simulink model "gm_gaussianFilter"  (R2024a)
settings: Solver=FixedStepDiscrete  StartTime=0.0  StopTime=1  RelTol=1e-3
undefined symbols (not defined in the file or in its folder): G
libraries: hdlsllib x33, simulink x27, visionsources x1, visionsinks x1
(part 2 of 2)

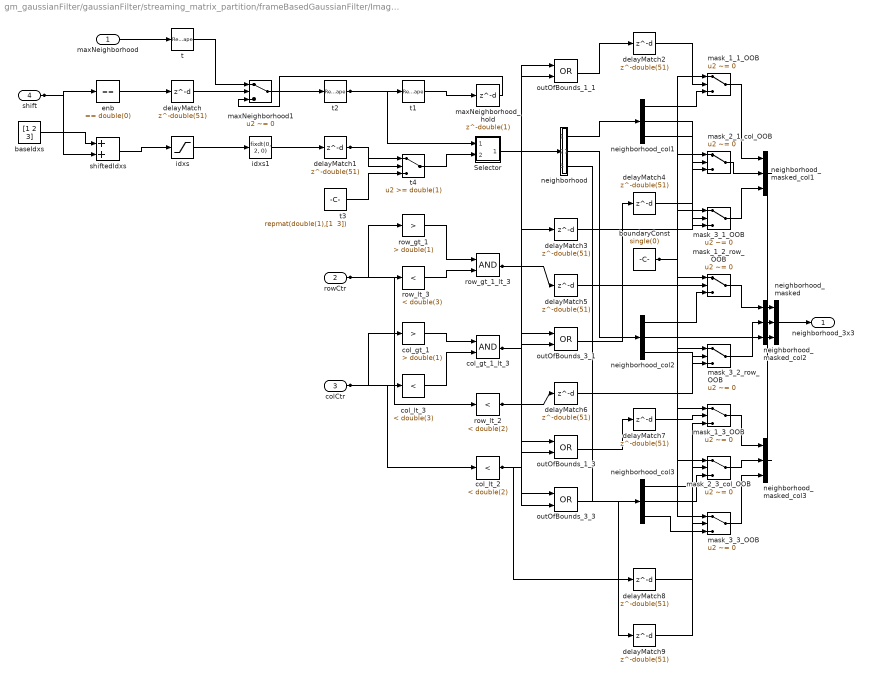
== system gm_gaussianFilter/gaussianFilter/streaming_matrix_partition/frameBasedGaussianFilter/ImageIn_NeighborhoodCreator/BoundaryCheck_3x3 ==
  maxNeighborhood : Inport  OutDataTypeStr=single  SampleTime=2.77039007092199e-06
  rowCtr : Inport  Port=2  OutDataTypeStr=fixdt(0,9,0,'DataTypeOverride', 'Off')  SampleTime=2.77039007092199e-06
  colCtr : Inport  Port=3  OutDataTypeStr=fixdt(0,10,0,'DataTypeOverride', 'Off')  SampleTime=2.77039007092199e-06
  shift : Inport  Port=4  OutDataTypeStr=fixdt(0,1,0,'DataTypeOverride', 'Off')  SampleTime=2.77039007092199e-06
  Selector : Subsystem
  baseIdxs : Constant  Value=[1 2 3]  OutDataTypeStr=fixdt(0, 2, 0)  SampleTime=2.77039007092199e-06
  boundaryConst : Constant  Value=single(0)  OutDataTypeStr=single  SampleTime=2.77039007092199e-06
  col_gt_1 : simulink/Logic and Bit Operations/Compare To Constant  relop=>  const=double(1)  OutDataTypeStr=boolean
  col_gt_1_lt_3 : Logic  AllPortsSameDT=off  OutDataTypeStr=boolean  SampleTime=2.77039007092199e-06
  col_lt_2 : simulink/Logic and Bit Operations/Compare To Constant  relop=<  const=double(2)  OutDataTypeStr=boolean
  col_lt_3 : simulink/Logic and Bit Operations/Compare To Constant  relop=<  const=double(3)  OutDataTypeStr=boolean
  delayMatch{,1..9} (10 alike) : Delay  DelayLength=double(51)  InitialCondition=0  SampleTime=2.77039007092199e-06
  enb : simulink/Logic and Bit Operations/Compare To Constant  relop===  const=double(0)  OutDataTypeStr=boolean
  idxs : Saturate  UpperLimit=double(3)  LowerLimit=double(1)  SampleTime=2.77039007092199e-06  OutDataTypeStr=fixdt(0, 3, 0)
  idxs1 : DataTypeConversion  OutDataTypeStr=fixdt(0, 2, 0)  SampleTime=2.77039007092199e-06  SaturateOnIntegerOverflow=off  RndMeth=Floor
  mask_1_1_OOB : Switch  Criteria=u2 ~= 0  Threshold=double(0)  OutDataTypeStr=single  SampleTime=2.77039007092199e-06  SaturateOnIntegerOverflow=off  InputSameDT=off
  mask_1_2_row_OOB : Switch  Criteria=u2 ~= 0  Threshold=double(0)  OutDataTypeStr=single  SampleTime=2.77039007092199e-06  SaturateOnIntegerOverflow=off  InputSameDT=off
  mask_1_3_OOB : Switch  Criteria=u2 ~= 0  Threshold=double(0)  OutDataTypeStr=single  SampleTime=2.77039007092199e-06  SaturateOnIntegerOverflow=off  InputSameDT=off
  mask_2_1_col_OOB : Switch  Criteria=u2 ~= 0  Threshold=double(0)  OutDataTypeStr=single  SampleTime=2.77039007092199e-06  SaturateOnIntegerOverflow=off  InputSameDT=off
  mask_2_3_col_OOB : Switch  Criteria=u2 ~= 0  Threshold=double(0)  OutDataTypeStr=single  SampleTime=2.77039007092199e-06  SaturateOnIntegerOverflow=off  InputSameDT=off
  mask_3_1_OOB : Switch  Criteria=u2 ~= 0  Threshold=double(0)  OutDataTypeStr=single  SampleTime=2.77039007092199e-06  SaturateOnIntegerOverflow=off  InputSameDT=off
  mask_3_2_row_OOB : Switch  Criteria=u2 ~= 0  Threshold=double(0)  OutDataTypeStr=single  SampleTime=2.77039007092199e-06  SaturateOnIntegerOverflow=off  InputSameDT=off
  mask_3_3_OOB : Switch  Criteria=u2 ~= 0  Threshold=double(0)  OutDataTypeStr=single  SampleTime=2.77039007092199e-06  SaturateOnIntegerOverflow=off  InputSameDT=off
  maxNeighborhood1 : Switch  Criteria=u2 ~= 0  Threshold=double(0)  OutDataTypeStr=single  SampleTime=2.77039007092199e-06  SaturateOnIntegerOverflow=off  InputSameDT=off
  maxNeighborhood_hold : Delay  DelayLength=double(1)  InitialCondition=0  SampleTime=2.77039007092199e-06
  neighborhood : Subsystem
  neighborhood_col1 : Demux  Outputs=3
  neighborhood_col2 : Demux  Outputs=3
  neighborhood_col3 : Demux  Outputs=3
  neighborhood_masked : Concatenate  NumInputs=3  Mode=Multidimensional array  ConcatenateDimension=2
  neighborhood_masked_col1 : Concatenate  NumInputs=3  Mode=Multidimensional array
  neighborhood_masked_col2 : Concatenate  NumInputs=3  Mode=Multidimensional array
  neighborhood_masked_col3 : Concatenate  NumInputs=3  Mode=Multidimensional array
  outOfBounds_1_1 : Logic  Operator=OR  AllPortsSameDT=off  OutDataTypeStr=boolean  SampleTime=2.77039007092199e-06
  outOfBounds_1_3 : Logic  Operator=OR  AllPortsSameDT=off  OutDataTypeStr=boolean  SampleTime=2.77039007092199e-06
  outOfBounds_3_1 : Logic  Operator=OR  AllPortsSameDT=off  OutDataTypeStr=boolean  SampleTime=2.77039007092199e-06
  outOfBounds_3_3 : Logic  Operator=OR  AllPortsSameDT=off  OutDataTypeStr=boolean  SampleTime=2.77039007092199e-06
  row_gt_1 : simulink/Logic and Bit Operations/Compare To Constant  relop=>  const=double(1)  OutDataTypeStr=boolean
  row_gt_1_lt_3 : Logic  AllPortsSameDT=off  OutDataTypeStr=boolean  SampleTime=2.77039007092199e-06
  row_lt_2 : simulink/Logic and Bit Operations/Compare To Constant  relop=<  const=double(2)  OutDataTypeStr=boolean
  row_lt_3 : simulink/Logic and Bit Operations/Compare To Constant  relop=<  const=double(3)  OutDataTypeStr=boolean
  shiftedIdxs : Sum  OutDataTypeStr=fixdt(0, 3, 0)  SampleTime=2.77039007092199e-06
  t : Reshape  OutputDimensionality=Column vector (2-D)
  t1 : Reshape  OutputDimensionality=Column vector (2-D)
  t2 : Reshape  OutputDimensionality=Customize  OutputDimensions=[3,3]
  t3 : Constant  Value="repmat(double(1),[1  3])"  OutDataTypeStr=fixdt(0, 2, 0)  SampleTime=2.77039007092199e-06
  t4 : Switch  Threshold=double(1)  OutDataTypeStr=fixdt(0, 2, 0)  SampleTime=2.77039007092199e-06  SaturateOnIntegerOverflow=off  InputSameDT=off
  neighborhood_3x3 : Outport  OutDataTypeStr=single  SampleTime=2.77039007092199e-06
  wires:
  maxNeighborhood/1 -> t/1
  rowCtr/1 -> row_lt_2/1, row_lt_3/1, row_gt_1/1
  colCtr/1 -> col_lt_2/1, col_lt_3/1, col_gt_1/1
  shift/1 -> shiftedIdxs/2, enb/1
  delayMatch/1 -> maxNeighborhood1/2
  baseIdxs/1 -> shiftedIdxs/1
  shiftedIdxs/1 -> idxs/1
  idxs/1 -> idxs1/1
  delayMatch1/1 -> t4/2, t4/1
  Selector/1(Out1) -> neighborhood/1(in0)
  boundaryConst/1 -> mask_3_3_OOB/1, mask_3_2_row_OOB/1, mask_3_1_OOB/1, mask_2_3_col_OOB/1, mask_2_1_col_OOB/1, mask_1_3_OOB/1, mask_1_2_row_OOB/1, mask_1_1_OOB/1
  neighborhood_col1/1 -> mask_1_1_OOB/3
  neighborhood_col2/1 -> mask_1_2_row_OOB/3
  neighborhood_col3/1 -> mask_1_3_OOB/3
  neighborhood_col1/2 -> mask_2_1_col_OOB/3
  neighborhood_col2/2 -> neighborhood_masked_col2/2
  neighborhood_col3/2 -> mask_2_3_col_OOB/3
  neighborhood_col1/3 -> mask_3_1_OOB/3
  neighborhood_col2/3 -> mask_3_2_row_OOB/3
  neighborhood_col3/3 -> mask_3_3_OOB/3
  neighborhood/1(out0) -> neighborhood_col1/1
  neighborhood/2(out1) -> neighborhood_col2/1
  neighborhood/3(out2) -> neighborhood_col3/1
  row_gt_1/1 -> row_gt_1_lt_3/1
  row_lt_3/1 -> row_gt_1_lt_3/2
  delayMatch5/1 -> mask_1_2_row_OOB/2
  col_gt_1/1 -> col_gt_1_lt_3/1
  col_lt_3/1 -> col_gt_1_lt_3/2
  delayMatch3/1 -> mask_2_1_col_OOB/2
  delayMatch2/1 -> mask_1_1_OOB/2
  mask_1_1_OOB/1 -> neighborhood_masked_col1/1
  mask_1_2_row_OOB/1 -> neighborhood_masked_col2/1
  delayMatch8/1 -> mask_2_3_col_OOB/2
  delayMatch7/1 -> mask_1_3_OOB/2
  mask_1_3_OOB/1 -> neighborhood_masked_col3/1
  mask_2_1_col_OOB/1 -> neighborhood_masked_col1/2
  mask_2_3_col_OOB/1 -> neighborhood_masked_col3/2
  delayMatch6/1 -> mask_3_2_row_OOB/2
  delayMatch4/1 -> mask_3_1_OOB/2
  mask_3_1_OOB/1 -> neighborhood_masked_col1/3
  mask_3_2_row_OOB/1 -> neighborhood_masked_col2/3
  delayMatch9/1 -> mask_3_3_OOB/2
  mask_3_3_OOB/1 -> neighborhood_masked_col3/3
  neighborhood_masked/1 -> neighborhood_3x3/1
  neighborhood_masked_col1/1 -> neighborhood_masked/1
  neighborhood_masked_col2/1 -> neighborhood_masked/2
  neighborhood_masked_col3/1 -> neighborhood_masked/3
  t/1 -> maxNeighborhood1/1
  enb/1 -> delayMatch/1
  idxs1/1 -> delayMatch1/1
  outOfBounds_1_1/1 -> delayMatch2/1
  col_gt_1_lt_3/1 -> delayMatch3/1, outOfBounds_3_1/2, outOfBounds_1_1/2
  outOfBounds_3_1/1 -> delayMatch4/1
  row_gt_1_lt_3/1 -> delayMatch5/1, outOfBounds_1_3/1, outOfBounds_1_1/1
  row_lt_2/1 -> delayMatch6/1, outOfBounds_3_3/1, outOfBounds_3_1/1
  outOfBounds_1_3/1 -> delayMatch7/1
  col_lt_2/1 -> delayMatch8/1, outOfBounds_3_3/2, outOfBounds_1_3/2
  outOfBounds_3_3/1 -> delayMatch9/1
  t2/1 -> t1/1, Selector/1(In1)
  t1/1 -> maxNeighborhood_hold/1
  maxNeighborhood_hold/1 -> maxNeighborhood1/3
  maxNeighborhood1/1 -> t2/1
  t3/1 -> t4/3
  t4/1 -> Selector/2(In2)

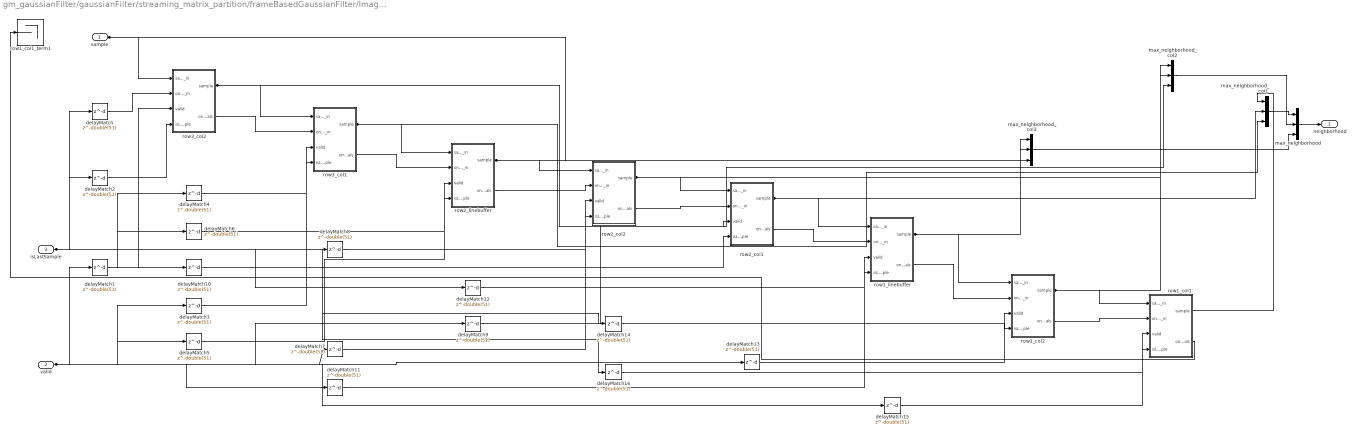
== system gm_gaussianFilter/gaussianFilter/streaming_matrix_partition/frameBasedGaussianFilter/ImageIn_NeighborhoodCreator/NeighborhoodCreator_3x3 ==
  sample : Inport  OutDataTypeStr=single  SampleTime=2.77039007092199e-06
  valid : Inport  Port=2  OutDataTypeStr=boolean  SampleTime=2.77039007092199e-06
  isLastSample : Inport  Port=3  OutDataTypeStr=boolean  SampleTime=2.77039007092199e-06
  delayMatch{,1..16} (17 alike) : Delay  DelayLength=double(51)  InitialCondition=0  SampleTime=2.77039007092199e-06
  max_neighborhood : Concatenate  NumInputs=3  Mode=Multidimensional array  ConcatenateDimension=2
  max_neighborhood_col1 : Concatenate  NumInputs=3  Mode=Multidimensional array
  max_neighborhood_col2 : Concatenate  NumInputs=3  Mode=Multidimensional array
  max_neighborhood_col3 : Concatenate  NumInputs=3  Mode=Multidimensional array
  row1_col1 : Subsystem
  row1_col1_term1 : Terminator
  row1_col2 : Subsystem
  row1_linebuffer : Subsystem
  row2_col1 : Subsystem
  row2_col2 : Subsystem
  row2_linebuffer : Subsystem
  row3_col1 : Subsystem
  row3_col2 : Subsystem
  neighborhood : Outport  OutDataTypeStr=single  SampleTime=2.77039007092199e-06
  wires:
  sample/1 -> max_neighborhood_col3/3, row3_col2/1(sample_in)
  delayMatch1/1 -> row3_col2/3(valid)
  delayMatch/1 -> row3_col2/2(onEndVals_in)
  row3_col2/1(sample) -> max_neighborhood_col2/3, row3_col1/1(sample_in)
  row3_col2/2(onEndVals) -> row3_col1/2(onEndVals_in)
  row3_col1/1(sample) -> max_neighborhood_col1/3, row2_linebuffer/1(sample_in)
  row3_col1/2(onEndVals) -> row2_linebuffer/2(onEndVals_in)
  row2_linebuffer/1(sample) -> max_neighborhood_col3/2, row2_col2/1(sample_in)
  row2_linebuffer/2(onEndVals) -> row2_col2/2(onEndVals_in)
  row2_col2/1(sample) -> max_neighborhood_col2/2, row2_col1/1(sample_in)
  row2_col2/2(onEndVals) -> row2_col1/2(onEndVals_in)
  row2_col1/1(sample) -> max_neighborhood_col1/2, row1_linebuffer/1(sample_in)
  row2_col1/2(onEndVals) -> row1_linebuffer/2(onEndVals_in)
  row1_linebuffer/1(sample) -> max_neighborhood_col3/1, row1_col2/1(sample_in)
  row1_linebuffer/2(onEndVals) -> row1_col2/2(onEndVals_in)
  row1_col2/1(sample) -> max_neighborhood_col2/1, row1_col1/1(sample_in)
  row1_col2/2(onEndVals) -> row1_col1/2(onEndVals_in)
  row1_col1/1(sample) -> max_neighborhood_col1/1
  row1_col1/2(onEndVals) -> row1_col1_term1/1
  max_neighborhood/1 -> neighborhood/1
  max_neighborhood_col1/1 -> max_neighborhood/1
  max_neighborhood_col2/1 -> max_neighborhood/2
  max_neighborhood_col3/1 -> max_neighborhood/3
  delayMatch2/1 -> row3_col2/4(isLastSample)
  delayMatch3/1 -> row3_col1/3(valid)
  delayMatch4/1 -> row3_col1/4(isLastSample)
  delayMatch5/1 -> row2_linebuffer/3(valid)
  delayMatch6/1 -> row2_linebuffer/4(isLastSample)
  delayMatch7/1 -> row2_col2/3(valid)
  delayMatch8/1 -> row2_col2/4(isLastSample)
  delayMatch9/1 -> row2_col1/3(valid)
  delayMatch10/1 -> row2_col1/4(isLastSample)
  delayMatch11/1 -> row1_linebuffer/3(valid)
  delayMatch12/1 -> row1_linebuffer/4(isLastSample)
  delayMatch13/1 -> row1_col2/3(valid)
  delayMatch14/1 -> row1_col2/4(isLastSample)
  delayMatch15/1 -> row1_col1/3(valid)
  delayMatch16/1 -> row1_col1/4(isLastSample)
  valid/1 -> delayMatch15/1, delayMatch13/1, delayMatch11/1, delayMatch9/1, delayMatch7/1, delayMatch5/1, delayMatch3/1, delayMatch1/1
  isLastSample/1 -> delayMatch16/1, delayMatch14/1, delayMatch12/1, delayMatch10/1, delayMatch8/1, delayMatch6/1, delayMatch4/1, delayMatch2/1, delayMatch/1

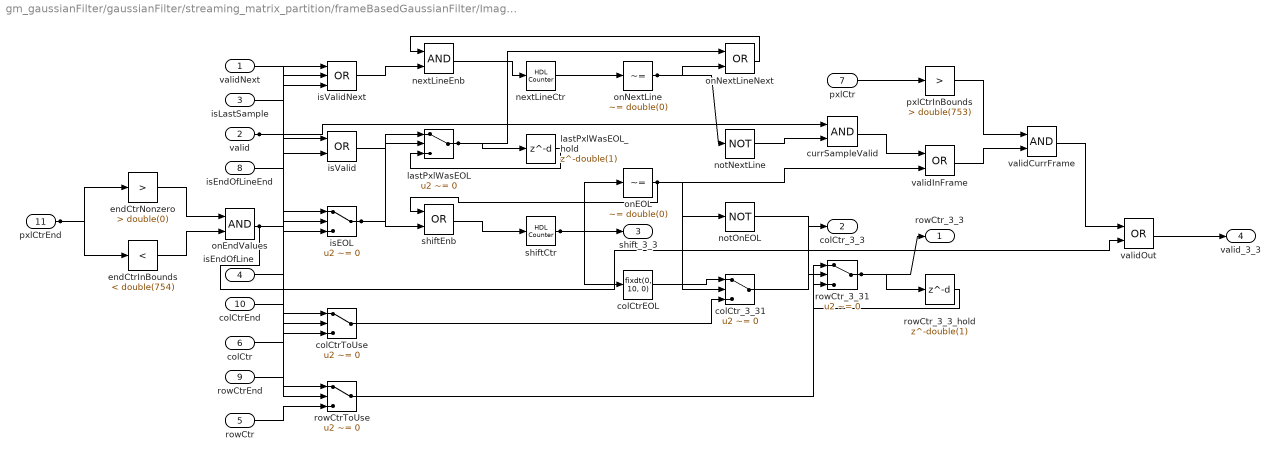
== system gm_gaussianFilter/gaussianFilter/streaming_matrix_partition/frameBasedGaussianFilter/ImageIn_NeighborhoodCreator/boundaryCounters_3_3 ==
  validNext : Inport  OutDataTypeStr=boolean  SampleTime=2.77039007092199e-06
  valid : Inport  Port=2  OutDataTypeStr=boolean  SampleTime=2.77039007092199e-06
  isLastSample : Inport  Port=3  OutDataTypeStr=boolean  SampleTime=2.77039007092199e-06
  isEndOfLine : Inport  Port=4  OutDataTypeStr=boolean  SampleTime=2.77039007092199e-06
  rowCtr : Inport  Port=5  OutDataTypeStr=fixdt(0,9,0,'DataTypeOverride', 'Off')  SampleTime=2.77039007092199e-06
  colCtr : Inport  Port=6  OutDataTypeStr=fixdt(0,10,0,'DataTypeOverride', 'Off')  SampleTime=2.77039007092199e-06
  pxlCtr : Inport  Port=7  OutDataTypeStr=fixdt(0,19,0,'DataTypeOverride', 'Off')  SampleTime=2.77039007092199e-06
  isEndOfLineEnd : Inport  Port=8  OutDataTypeStr=boolean  SampleTime=2.77039007092199e-06
  rowCtrEnd : Inport  Port=9  OutDataTypeStr=fixdt(0,9,0,'DataTypeOverride', 'Off')  SampleTime=2.77039007092199e-06
  colCtrEnd : Inport  Port=10  OutDataTypeStr=fixdt(0,10,0,'DataTypeOverride', 'Off')  SampleTime=2.77039007092199e-06
  pxlCtrEnd : Inport  Port=11  OutDataTypeStr=fixdt(0,19,0,'DataTypeOverride', 'Off')  SampleTime=2.77039007092199e-06
  colCtrEOL : DataTypeConversion  OutDataTypeStr=fixdt(0, 10, 0)  SampleTime=2.77039007092199e-06  SaturateOnIntegerOverflow=off  RndMeth=Floor
  colCtrToUse : Switch  Criteria=u2 ~= 0  Threshold=double(0)  OutDataTypeStr=fixdt(0, 10, 0)  SampleTime=2.77039007092199e-06  SaturateOnIntegerOverflow=off  InputSameDT=off
  colCtr_3_31 : Switch  Criteria=u2 ~= 0  Threshold=double(0)  OutDataTypeStr=fixdt(0, 10, 0)  SampleTime=2.77039007092199e-06  SaturateOnIntegerOverflow=off  InputSameDT=off
  currSampleValid : Logic  AllPortsSameDT=off  OutDataTypeStr=boolean  SampleTime=2.77039007092199e-06
  endCtrInBounds : simulink/Logic and Bit Operations/Compare To Constant  relop=<  const=double(754)  OutDataTypeStr=boolean
  endCtrNonzero : simulink/Logic and Bit Operations/Compare To Constant  relop=>  const=double(0)  OutDataTypeStr=boolean
  isEOL : Switch  Criteria=u2 ~= 0  Threshold=double(0)  OutDataTypeStr=boolean  SampleTime=2.77039007092199e-06  SaturateOnIntegerOverflow=off  InputSameDT=off
  isValid : Logic  Operator=OR  AllPortsSameDT=off  OutDataTypeStr=boolean  SampleTime=2.77039007092199e-06
  isValidNext : Logic  Operator=OR  Inputs=3  AllPortsSameDT=off  OutDataTypeStr=boolean  SampleTime=2.77039007092199e-06
  lastPxlWasEOL : Switch  Criteria=u2 ~= 0  Threshold=double(0)  OutDataTypeStr=boolean  SampleTime=2.77039007092199e-06  SaturateOnIntegerOverflow=off  InputSameDT=off
  lastPxlWasEOL_hold : Delay  DelayLength=double(1)  InitialCondition=0  SampleTime=2.77039007092199e-06
  nextLineCtr : hdlsllib/Sources/HDL Counter  CountType=Count limited  CountInit=double(0)  CountStep=double(1)  CountMax=double(1)  CountFromType=Initial value  CountFrom=double(0)  CountResetPort=off  CountLoadPort=off  CountEnbPort=on  CountDirPort=off  CountHitOutputPort=off  CountDataType=Unsigned  CountWordLen=1  CountFracLen=0  CountSampTime=2.77039007092199e-06
  nextLineEnb : Logic  AllPortsSameDT=off  OutDataTypeStr=boolean  SampleTime=2.77039007092199e-06
  notNextLine : Logic  Operator=NOT  Inputs=1  AllPortsSameDT=off  OutDataTypeStr=boolean  SampleTime=2.77039007092199e-06
  notOnEOL : Logic  Operator=NOT  Inputs=1  AllPortsSameDT=off  OutDataTypeStr=boolean  SampleTime=2.77039007092199e-06
  onEOL : simulink/Logic and Bit Operations/Compare To Constant  relop=~=  const=double(0)  OutDataTypeStr=boolean
  onEndValues : Logic  AllPortsSameDT=off  OutDataTypeStr=boolean  SampleTime=2.77039007092199e-06
  onNextLine : simulink/Logic and Bit Operations/Compare To Constant  relop=~=  const=double(0)  OutDataTypeStr=boolean
  onNextLineNext : Logic  Operator=OR  AllPortsSameDT=off  OutDataTypeStr=boolean  SampleTime=2.77039007092199e-06
  pxlCtrInBounds : simulink/Logic and Bit Operations/Compare To Constant  relop=>  const=double(753)  OutDataTypeStr=boolean
  rowCtrToUse : Switch  Criteria=u2 ~= 0  Threshold=double(0)  OutDataTypeStr=fixdt(0, 9, 0)  SampleTime=2.77039007092199e-06  SaturateOnIntegerOverflow=off  InputSameDT=off
  rowCtr_3_31 : Switch  Criteria=u2 ~= 0  Threshold=double(0)  OutDataTypeStr=fixdt(0, 9, 0)  SampleTime=2.77039007092199e-06  SaturateOnIntegerOverflow=off  InputSameDT=off
  rowCtr_3_3_hold : Delay  DelayLength=double(1)  InitialCondition=0  SampleTime=2.77039007092199e-06
  shiftCtr : hdlsllib/Sources/HDL Counter  CountType=Count limited  CountInit=double(0)  CountStep=double(1)  CountMax=double(1)  CountFromType=Initial value  CountFrom=double(0)  CountResetPort=off  CountLoadPort=off  CountEnbPort=on  CountDirPort=off  CountHitOutputPort=off  CountDataType=Unsigned  CountWordLen=1  CountFracLen=0  CountSampTime=2.77039007092199e-06
  shiftEnb : Logic  Operator=OR  AllPortsSameDT=off  OutDataTypeStr=boolean  SampleTime=2.77039007092199e-06
  validCurrFrame : Logic  AllPortsSameDT=off  OutDataTypeStr=boolean  SampleTime=2.77039007092199e-06
  validInFrame : Logic  Operator=OR  AllPortsSameDT=off  OutDataTypeStr=boolean  SampleTime=2.77039007092199e-06
  validOut : Logic  Operator=OR  AllPortsSameDT=off  OutDataTypeStr=boolean  SampleTime=2.77039007092199e-06
  rowCtr_3_3 : Outport  OutDataTypeStr=fixdt(0,9,0,'DataTypeOverride', 'Off')  SampleTime=2.77039007092199e-06
  colCtr_3_3 : Outport  Port=2  OutDataTypeStr=fixdt(0,10,0,'DataTypeOverride', 'Off')  SampleTime=2.77039007092199e-06
  shift_3_3 : Outport  Port=3  OutDataTypeStr=fixdt(0,1,0,'DataTypeOverride', 'Off')  SampleTime=2.77039007092199e-06
  valid_3_3 : Outport  Port=4  OutDataTypeStr=boolean  SampleTime=2.77039007092199e-06
  wires:
  validNext/1 -> isValidNext/2
  valid/1 -> currSampleValid/1, isValid/2
  isLastSample/1 -> isValidNext/3
  isEndOfLine/1 -> isEOL/3
  rowCtr/1 -> rowCtrToUse/3
  colCtr/1 -> colCtrToUse/3
  pxlCtr/1 -> pxlCtrInBounds/1
  isEndOfLineEnd/1 -> isEOL/1
  rowCtrEnd/1 -> rowCtrToUse/1
  colCtrEnd/1 -> colCtrToUse/1
  pxlCtrEnd/1 -> endCtrInBounds/1, endCtrNonzero/1
  endCtrNonzero/1 -> onEndValues/1
  endCtrInBounds/1 -> onEndValues/2
  onEndValues/1 -> validOut/2, isValidNext/1, isEOL/2, isValid/1, colCtrToUse/2, rowCtrToUse/2
  rowCtrToUse/1 -> rowCtr_3_31/1
  colCtrToUse/1 -> colCtr_3_31/3
  isValid/1 -> lastPxlWasEOL/2
  isEOL/1 -> shiftEnb/2, lastPxlWasEOL/1
  isValidNext/1 -> nextLineEnb/2
  shiftCtr/1 -> shift_3_3/1, colCtrEOL/1, onEOL/1
  onEOL/1 -> validInFrame/2, colCtr_3_31/2, notOnEOL/1, shiftEnb/1
  lastPxlWasEOL/1 -> lastPxlWasEOL_hold/1, onNextLineNext/1
  onNextLine/1 -> notNextLine/1, onNextLineNext/2
  notOnEOL/1 -> rowCtr_3_31/2
  rowCtr_3_31/1 -> rowCtr_3_3/1, rowCtr_3_3_hold/1
  colCtrEOL/1 -> colCtr_3_31/1
  colCtr_3_31/1 -> colCtr_3_3/1
  notNextLine/1 -> currSampleValid/2
  currSampleValid/1 -> validInFrame/1
  validInFrame/1 -> validCurrFrame/2
  pxlCtrInBounds/1 -> validCurrFrame/1
  validCurrFrame/1 -> validOut/1
  validOut/1 -> valid_3_3/1
  shiftEnb/1 -> shiftCtr/1
  rowCtr_3_3_hold/1 -> rowCtr_3_31/3
  lastPxlWasEOL_hold/1 -> lastPxlWasEOL/3
  onNextLineNext/1 -> nextLineEnb/1
  nextLineEnb/1 -> nextLineCtr/1
  nextLineCtr/1 -> onNextLine/1

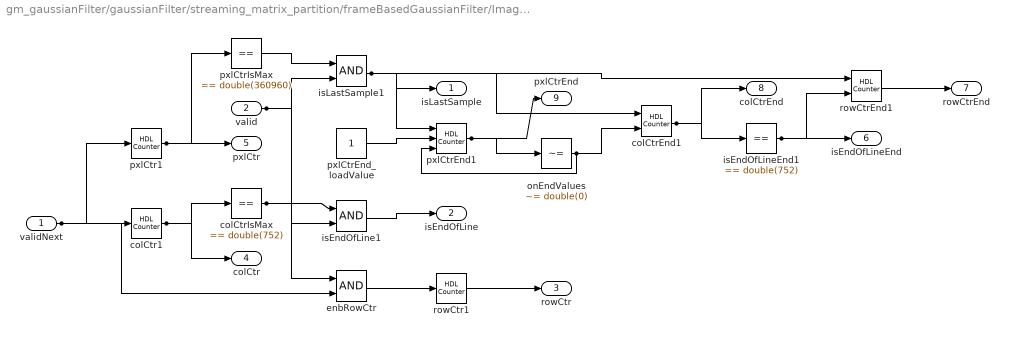
== system gm_gaussianFilter/gaussianFilter/streaming_matrix_partition/frameBasedGaussianFilter/ImageIn_NeighborhoodCreator/counterNetwork ==
  validNext : Inport  OutDataTypeStr=boolean  SampleTime=2.77039007092199e-06
  valid : Inport  Port=2  OutDataTypeStr=boolean  SampleTime=2.77039007092199e-06
  colCtr1 : hdlsllib/Sources/HDL Counter  CountType=Count limited  CountInit=double(752)  CountStep=double(1)  CountMax=double(752)  CountFromType=Specify  CountFrom=double(1)  CountResetPort=off  CountLoadPort=off  CountEnbPort=on  CountDirPort=off  CountHitOutputPort=off  CountDataType=Unsigned  CountWordLen=10  CountFracLen=0  CountSampTime=2.77039007092199e-06
  colCtrEnd1 : hdlsllib/Sources/HDL Counter  CountType=Count limited  CountInit=double(1)  CountStep=double(1)  CountMax=double(752)  CountFromType=Initial value  CountFrom=double(1)  CountResetPort=on  CountLoadPort=off  CountEnbPort=on  CountDirPort=off  CountHitOutputPort=off  CountDataType=Unsigned  CountWordLen=10  CountFracLen=0  CountSampTime=2.77039007092199e-06
  colCtrIsMax : simulink/Logic and Bit Operations/Compare To Constant  relop===  const=double(752)  OutDataTypeStr=boolean
  enbRowCtr : Logic  AllPortsSameDT=off  OutDataTypeStr=boolean  SampleTime=2.77039007092199e-06
  isEndOfLine1 : Logic  AllPortsSameDT=off  OutDataTypeStr=boolean  SampleTime=2.77039007092199e-06
  isEndOfLineEnd1 : simulink/Logic and Bit Operations/Compare To Constant  relop===  const=double(752)  OutDataTypeStr=boolean
  isLastSample1 : Logic  AllPortsSameDT=off  OutDataTypeStr=boolean  SampleTime=2.77039007092199e-06
  onEndValues : simulink/Logic and Bit Operations/Compare To Constant  relop=~=  const=double(0)  OutDataTypeStr=boolean
  pxlCtr1 : hdlsllib/Sources/HDL Counter  CountType=Count limited  CountInit=double(360960)  CountStep=double(1)  CountMax=double(360960)  CountFromType=Specify  CountFrom=double(1)  CountResetPort=off  CountLoadPort=off  CountEnbPort=on  CountDirPort=off  CountHitOutputPort=off  CountDataType=Unsigned  CountWordLen=19  CountFracLen=0  CountSampTime=2.77039007092199e-06
  pxlCtrEnd1 : hdlsllib/Sources/HDL Counter  CountType=Count limited  CountInit=double(0)  CountStep=double(1)  CountMax=double(1507)  CountFromType=Initial value  CountFrom=double(0)  CountResetPort=off  CountLoadPort=on  CountEnbPort=on  CountDirPort=off  CountHitOutputPort=off  CountDataType=Unsigned  CountWordLen=19  CountFracLen=0  CountSampTime=2.77039007092199e-06
  pxlCtrEnd_loadValue : Constant  OutDataTypeStr=fixdt(0, 19, 0)  SampleTime=2.77039007092199e-06
  pxlCtrIsMax : simulink/Logic and Bit Operations/Compare To Constant  relop===  const=double(360960)  OutDataTypeStr=boolean
  rowCtr1 : hdlsllib/Sources/HDL Counter  CountType=Count limited  CountInit=double(480)  CountStep=double(1)  CountMax=double(480)  CountFromType=Specify  CountFrom=double(1)  CountResetPort=off  CountLoadPort=off  CountEnbPort=on  CountDirPort=off  CountHitOutputPort=off  CountDataType=Unsigned  CountWordLen=9  CountFracLen=0  CountSampTime=2.77039007092199e-06
  rowCtrEnd1 : hdlsllib/Sources/HDL Counter  CountType=Count limited  CountInit=double(1)  CountStep=double(1)  CountMax=double(480)  CountFromType=Initial value  CountFrom=double(1)  CountResetPort=on  CountLoadPort=off  CountEnbPort=on  CountDirPort=off  CountHitOutputPort=off  CountDataType=Unsigned  CountWordLen=9  CountFracLen=0  CountSampTime=2.77039007092199e-06
  isLastSample : Outport  OutDataTypeStr=boolean  SampleTime=2.77039007092199e-06
  isEndOfLine : Outport  Port=2  OutDataTypeStr=boolean  SampleTime=2.77039007092199e-06
  rowCtr : Outport  Port=3  OutDataTypeStr=fixdt(0,9,0,'DataTypeOverride', 'Off')  SampleTime=2.77039007092199e-06
  colCtr : Outport  Port=4  OutDataTypeStr=fixdt(0,10,0,'DataTypeOverride', 'Off')  SampleTime=2.77039007092199e-06
  pxlCtr : Outport  Port=5  OutDataTypeStr=fixdt(0,19,0,'DataTypeOverride', 'Off')  SampleTime=2.77039007092199e-06
  isEndOfLineEnd : Outport  Port=6  OutDataTypeStr=boolean  SampleTime=2.77039007092199e-06
  rowCtrEnd : Outport  Port=7  OutDataTypeStr=fixdt(0,9,0,'DataTypeOverride', 'Off')  SampleTime=2.77039007092199e-06
  colCtrEnd : Outport  Port=8  OutDataTypeStr=fixdt(0,10,0,'DataTypeOverride', 'Off')  SampleTime=2.77039007092199e-06
  pxlCtrEnd : Outport  Port=9  OutDataTypeStr=fixdt(0,19,0,'DataTypeOverride', 'Off')  SampleTime=2.77039007092199e-06
  wires:
  validNext/1 -> enbRowCtr/2, colCtr1/1, pxlCtr1/1
  valid/1 -> isEndOfLine1/2, isLastSample1/2
  pxlCtr1/1 -> pxlCtr/1, pxlCtrIsMax/1
  pxlCtrIsMax/1 -> isLastSample1/1
  isLastSample1/1 -> isLastSample/1, rowCtrEnd1/1, colCtrEnd1/1, pxlCtrEnd1/1
  pxlCtrEnd1/1 -> pxlCtrEnd/1, onEndValues/1
  onEndValues/1 -> colCtrEnd1/2, pxlCtrEnd1/3
  pxlCtrEnd_loadValue/1 -> pxlCtrEnd1/2
  colCtr1/1 -> colCtr/1, colCtrIsMax/1
  colCtrIsMax/1 -> isEndOfLine1/1, enbRowCtr/1
  enbRowCtr/1 -> rowCtr1/1
  rowCtr1/1 -> rowCtr/1
  isEndOfLine1/1 -> isEndOfLine/1
  colCtrEnd1/1 -> colCtrEnd/1, isEndOfLineEnd1/1
  isEndOfLineEnd1/1 -> isEndOfLineEnd/1, rowCtrEnd1/2
  rowCtrEnd1/1 -> rowCtrEnd/1

== system gm_gaussianFilter/gaussianFilter/streaming_matrix_partition/frameBasedGaussianFilter/gaussianKernel/multiplier ==
  In1 : Inport
  In2 : Inport  Port=2
  multiplier : Product  Inputs=**  OutDataTypeStr=single  SampleTime=2.77039007092199e-06
  multiplier_pd1 : Delay  DelayLength=6
  Out1 : Outport
  wires:
  In1/1 -> multiplier/1
  In2/1 -> multiplier/2
  multiplier/1 -> multiplier_pd1/1
  multiplier_pd1/1 -> Out1/1

== system gm_gaussianFilter/gaussianFilter/streaming_matrix_partition/frameBasedGaussianFilter/gaussianKernel/sum_stage2 ==
  In1 : Inport
  In2 : Inport  Port=2
  sum_stage2 : Sum  OutDataTypeStr=single  SampleTime=2.77039007092199e-06
  sum_stage2_pd1 : Delay  DelayLength=6
  Out1 : Outport
  wires:
  In1/1 -> sum_stage2/1
  In2/1 -> sum_stage2/2
  sum_stage2/1 -> sum_stage2_pd1/1
  sum_stage2_pd1/1 -> Out1/1

== system gm_gaussianFilter/gaussianFilter/streaming_matrix_partition/frameBasedGaussianFilter/gaussianKernel/sum_stage21 ==
  In1 : Inport
  In2 : Inport  Port=2
  sum_stage21 : Sum  OutDataTypeStr=single  SampleTime=2.77039007092199e-06
  sum_stage21_pd1 : Delay  DelayLength=6
  Out1 : Outport
  wires:
  In1/1 -> sum_stage21/1
  In2/1 -> sum_stage21/2
  sum_stage21/1 -> sum_stage21_pd1/1
  sum_stage21_pd1/1 -> Out1/1

== system gm_gaussianFilter/gaussianFilter/streaming_matrix_partition/frameBasedGaussianFilter/gaussianKernel/sum_stage22 ==
  In1 : Inport
  In2 : Inport  Port=2
  sum_stage22 : Sum  OutDataTypeStr=single  SampleTime=2.77039007092199e-06
  sum_stage22_pd1 : Delay  DelayLength=6
  Out1 : Outport
  wires:
  In1/1 -> sum_stage22/1
  In2/1 -> sum_stage22/2
  sum_stage22/1 -> sum_stage22_pd1/1
  sum_stage22_pd1/1 -> Out1/1

== system gm_gaussianFilter/gaussianFilter/streaming_matrix_partition/frameBasedGaussianFilter/gaussianKernel/sum_stage23 ==
  In1 : Inport
  In2 : Inport  Port=2
  sum_stage23 : Sum  OutDataTypeStr=single  SampleTime=2.77039007092199e-06
  sum_stage23_pd1 : Delay  DelayLength=6
  Out1 : Outport
  wires:
  In1/1 -> sum_stage23/1
  In2/1 -> sum_stage23/2
  sum_stage23/1 -> sum_stage23_pd1/1
  sum_stage23_pd1/1 -> Out1/1

== system gm_gaussianFilter/gaussianFilter/streaming_matrix_partition/frameBasedGaussianFilter/gaussianKernel/sum_stage3 ==
  In1 : Inport
  In2 : Inport  Port=2
  sum_stage3 : Sum  OutDataTypeStr=single  SampleTime=2.77039007092199e-06
  sum_stage3_pd1 : Delay  DelayLength=6
  Out1 : Outport
  wires:
  In1/1 -> sum_stage3/1
  In2/1 -> sum_stage3/2
  sum_stage3/1 -> sum_stage3_pd1/1
  sum_stage3_pd1/1 -> Out1/1

== system gm_gaussianFilter/gaussianFilter/streaming_matrix_partition/frameBasedGaussianFilter/gaussianKernel/sum_stage31 ==
  In1 : Inport
  In2 : Inport  Port=2
  sum_stage31 : Sum  OutDataTypeStr=single  SampleTime=2.77039007092199e-06
  sum_stage31_pd1 : Delay  DelayLength=6
  Out1 : Outport
  wires:
  In1/1 -> sum_stage31/1
  In2/1 -> sum_stage31/2
  sum_stage31/1 -> sum_stage31_pd1/1
  sum_stage31_pd1/1 -> Out1/1

== system gm_gaussianFilter/gaussianFilter/streaming_matrix_partition/frameBasedGaussianFilter/gaussianKernel/sum_stage32 ==
  In1 : Inport
  In2 : Inport  Port=2
  sum_stage32 : Sum  OutDataTypeStr=single  SampleTime=2.77039007092199e-06
  sum_stage32_pd1 : Delay  DelayLength=6
  Out1 : Outport
  wires:
  In1/1 -> sum_stage32/1
  In2/1 -> sum_stage32/2
  sum_stage32/1 -> sum_stage32_pd1/1
  sum_stage32_pd1/1 -> Out1/1

== system gm_gaussianFilter/gaussianFilter/streaming_matrix_partition/frameBasedGaussianFilter/gaussianKernel/sum_stage33 ==
  In1 : Inport
  In2 : Inport  Port=2
  sum_stage33 : Sum  OutDataTypeStr=single  SampleTime=2.77039007092199e-06
  sum_stage33_pd1 : Delay  DelayLength=6
  Out1 : Outport
  wires:
  In1/1 -> sum_stage33/1
  In2/1 -> sum_stage33/2
  sum_stage33/1 -> sum_stage33_pd1/1
  sum_stage33_pd1/1 -> Out1/1

== system gm_gaussianFilter/gaussianFilter/streaming_matrix_partition/frameBasedGaussianFilter/gaussianKernel/t3 ==
  in0 : Inport
  ColVec1 : Selector  NumberOfDimensions=2  IndexOptions=Select all,Index vector (dialog)  Indices=1,1  OutputSizes=1,1
  ColVec2 : Selector  NumberOfDimensions=2  IndexOptions=Select all,Index vector (dialog)  Indices=1,2  OutputSizes=1,1
  ColVec3 : Selector  NumberOfDimensions=2  IndexOptions=Select all,Index vector (dialog)  Indices=1,3  OutputSizes=1,1
  out0 : Outport
  out1 : Outport  Port=2
  out2 : Outport  Port=3
  wires:
  in0/1 -> ColVec1/1, ColVec2/1, ColVec3/1
  ColVec1/1 -> out0/1
  ColVec2/1 -> out1/1
  ColVec3/1 -> out2/1

== system gm_gaussianFilter/gaussianFilter/streaming_matrix_partition/frameBasedGaussianFilter/ImageIn_NeighborhoodCreator/BoundaryCheck_3x3/Selector ==
  In1 : Inport
  In2 : Inport  Port=2
  Selector : Selector  NumberOfDimensions=2  IndexOptions=Select all,Index vector (port)  Indices=double(0),double(0)  OutputSizes=double(0),double(0)
  Selector_to_int2 : DataTypeConversion  OutDataTypeStr=uint32
  Out1 : Outport
  wires:
  In2/1 -> Selector_to_int2/1
  Selector_to_int2/1 -> Selector/2
  In1/1 -> Selector/1
  Selector/1 -> Out1/1

== system gm_gaussianFilter/gaussianFilter/streaming_matrix_partition/frameBasedGaussianFilter/ImageIn_NeighborhoodCreator/BoundaryCheck_3x3/neighborhood ==
  in0 : Inport
  ColVec1 : Selector  NumberOfDimensions=2  IndexOptions=Select all,Index vector (dialog)  Indices=1,1  OutputSizes=1,1
  ColVec2 : Selector  NumberOfDimensions=2  IndexOptions=Select all,Index vector (dialog)  Indices=1,2  OutputSizes=1,1
  ColVec3 : Selector  NumberOfDimensions=2  IndexOptions=Select all,Index vector (dialog)  Indices=1,3  OutputSizes=1,1
  out0 : Outport
  out1 : Outport  Port=2
  out2 : Outport  Port=3
  wires:
  in0/1 -> ColVec1/1, ColVec2/1, ColVec3/1
  ColVec1/1 -> out0/1
  ColVec2/1 -> out1/1
  ColVec3/1 -> out2/1

== system gm_gaussianFilter/gaussianFilter/streaming_matrix_partition/frameBasedGaussianFilter/ImageIn_NeighborhoodCreator/NeighborhoodCreator_3x3/row1_col1 ==
  sample_in : Inport  OutDataTypeStr=single  SampleTime=2.77039007092199e-06
  onEndVals_in : Inport  Port=2  OutDataTypeStr=boolean  SampleTime=2.77039007092199e-06
  valid : Inport  Port=3  OutDataTypeStr=boolean  SampleTime=2.77039007092199e-06
  isLastSample : Inport  Port=4  OutDataTypeStr=boolean  SampleTime=2.77039007092199e-06
  enb : Logic  Operator=OR  AllPortsSameDT=off  OutDataTypeStr=boolean  SampleTime=2.77039007092199e-06
  onEndVals1 : Logic  Operator=OR  AllPortsSameDT=off  OutDataTypeStr=boolean  SampleTime=2.77039007092199e-06
  onEndVals_delay : Delay  DelayLength=double(1)  InitialCondition=0  SampleTime=2.77039007092199e-06
  sample_delayed : Delay  DelayLength=double(1)  InitialCondition=double(0)  ShowEnablePort=on
      settings: InputPortMap=u0,e6
  sample : Outport  OutDataTypeStr=single  SampleTime=2.77039007092199e-06
  onEndVals : Outport  Port=2  OutDataTypeStr=boolean  SampleTime=2.77039007092199e-06
  wires:
  sample_in/1 -> sample_delayed/1
  onEndVals_in/1 -> onEndVals1/1
  valid/1 -> enb/1
  isLastSample/1 -> onEndVals1/2
  onEndVals1/1 -> onEndVals_delay/1
  onEndVals_delay/1 -> onEndVals/1, enb/2
  enb/1 -> sample_delayed/2
  sample_delayed/1 -> sample/1

== system gm_gaussianFilter/gaussianFilter/streaming_matrix_partition/frameBasedGaussianFilter/ImageIn_NeighborhoodCreator/NeighborhoodCreator_3x3/row1_col2 ==
  sample_in : Inport  OutDataTypeStr=single  SampleTime=2.77039007092199e-06
  onEndVals_in : Inport  Port=2  OutDataTypeStr=boolean  SampleTime=2.77039007092199e-06
  valid : Inport  Port=3  OutDataTypeStr=boolean  SampleTime=2.77039007092199e-06
  isLastSample : Inport  Port=4  OutDataTypeStr=boolean  SampleTime=2.77039007092199e-06
  enb : Logic  Operator=OR  AllPortsSameDT=off  OutDataTypeStr=boolean  SampleTime=2.77039007092199e-06
  onEndVals1 : Logic  Operator=OR  AllPortsSameDT=off  OutDataTypeStr=boolean  SampleTime=2.77039007092199e-06
  onEndVals_delay : Delay  DelayLength=double(1)  InitialCondition=0  SampleTime=2.77039007092199e-06
  sample_delayed : Delay  DelayLength=double(1)  InitialCondition=double(0)  ShowEnablePort=on
      settings: InputPortMap=u0,e6
  sample : Outport  OutDataTypeStr=single  SampleTime=2.77039007092199e-06
  onEndVals : Outport  Port=2  OutDataTypeStr=boolean  SampleTime=2.77039007092199e-06
  wires:
  sample_in/1 -> sample_delayed/1
  onEndVals_in/1 -> onEndVals1/1
  valid/1 -> enb/1
  isLastSample/1 -> onEndVals1/2
  onEndVals1/1 -> onEndVals_delay/1
  onEndVals_delay/1 -> onEndVals/1, enb/2
  enb/1 -> sample_delayed/2
  sample_delayed/1 -> sample/1

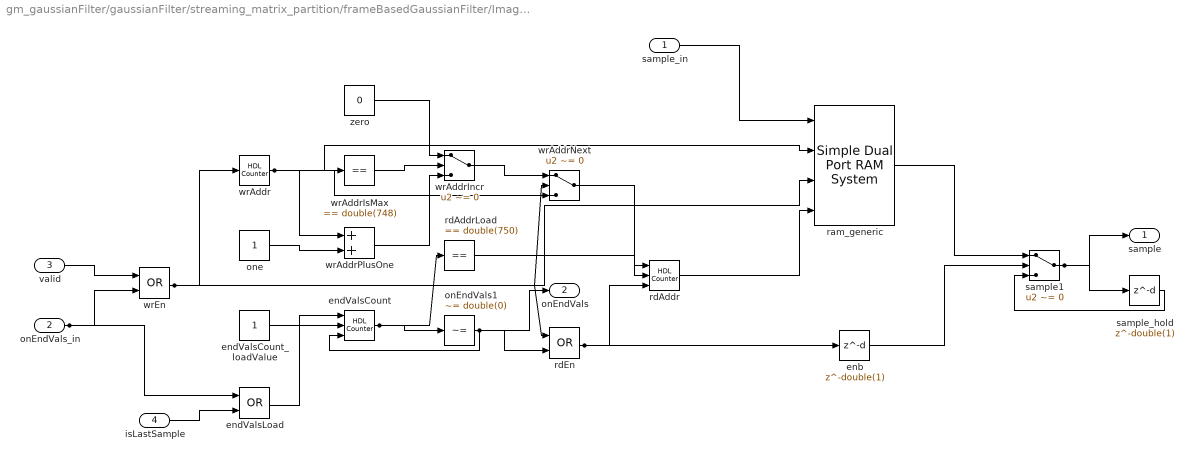
== system gm_gaussianFilter/gaussianFilter/streaming_matrix_partition/frameBasedGaussianFilter/ImageIn_NeighborhoodCreator/NeighborhoodCreator_3x3/row1_linebuffer ==
  sample_in : Inport  OutDataTypeStr=single  SampleTime=2.77039007092199e-06
  onEndVals_in : Inport  Port=2  OutDataTypeStr=boolean  SampleTime=2.77039007092199e-06
  valid : Inport  Port=3  OutDataTypeStr=boolean  SampleTime=2.77039007092199e-06
  isLastSample : Inport  Port=4  OutDataTypeStr=boolean  SampleTime=2.77039007092199e-06
  enb : Delay  DelayLength=double(1)  InitialCondition=0  SampleTime=2.77039007092199e-06
  endValsCount : hdlsllib/Sources/HDL Counter  CountType=Count limited  CountInit=double(0)  CountStep=double(1)  CountMax=double(750)  CountFromType=Initial value  CountFrom=double(0)  CountResetPort=off  CountLoadPort=on  CountEnbPort=on  CountDirPort=off  CountHitOutputPort=off  CountDataType=Unsigned  CountWordLen=10  CountFracLen=0  CountSampTime=2.77039007092199e-06
  endValsCount_loadValue : Constant  OutDataTypeStr=fixdt(0, 10, 0)  SampleTime=2.77039007092199e-06
  endValsLoad : Logic  Operator=OR  AllPortsSameDT=off  OutDataTypeStr=boolean  SampleTime=2.77039007092199e-06
  onEndVals1 : simulink/Logic and Bit Operations/Compare To Constant  relop=~=  const=double(0)  OutDataTypeStr=boolean
  one : Constant  OutDataTypeStr=fixdt(0, 10, 0)  SampleTime=2.77039007092199e-06
  ram_generic : hdlsllib/HDL RAMs/Simple Dual Port RAM System  RAMType=Simple dual port  AsyncRead=off  WriteOutputValue=New data  RAMInitialValue=0  allowBusInputs=off  WritesHaveOutput=on  NumReads=0  NumWrites=1  SimulateUsing=Code generation
  rdAddr : hdlsllib/Sources/HDL Counter  CountType=Count limited  CountInit=double(0)  CountStep=double(1)  CountMax=double(748)  CountFromType=Initial value  CountFrom=double(0)  CountResetPort=off  CountLoadPort=on  CountEnbPort=on  CountDirPort=off  CountHitOutputPort=off  CountDataType=Unsigned  CountWordLen=10  CountFracLen=0  CountSampTime=2.77039007092199e-06
  rdAddrLoad : simulink/Logic and Bit Operations/Compare To Constant  relop===  const=double(750)  OutDataTypeStr=boolean
  rdEn : Logic  Operator=OR  AllPortsSameDT=off  OutDataTypeStr=boolean  SampleTime=2.77039007092199e-06
  sample1 : Switch  Criteria=u2 ~= 0  Threshold=double(0)  OutDataTypeStr=single  SampleTime=2.77039007092199e-06  SaturateOnIntegerOverflow=off  InputSameDT=off
  sample_hold : Delay  DelayLength=double(1)  InitialCondition=0  SampleTime=2.77039007092199e-06
  wrAddr : hdlsllib/Sources/HDL Counter  CountType=Count limited  CountInit=double(0)  CountStep=double(1)  CountMax=double(748)  CountFromType=Initial value  CountFrom=double(0)  CountResetPort=off  CountLoadPort=off  CountEnbPort=on  CountDirPort=off  CountHitOutputPort=off  CountDataType=Unsigned  CountWordLen=10  CountFracLen=0  CountSampTime=2.77039007092199e-06
  wrAddrIncr : Switch  Criteria=u2 ~= 0  Threshold=double(0)  OutDataTypeStr=fixdt(0, 10, 0)  SampleTime=2.77039007092199e-06  SaturateOnIntegerOverflow=off  InputSameDT=off
  wrAddrIsMax : simulink/Logic and Bit Operations/Compare To Constant  relop===  const=double(748)  OutDataTypeStr=boolean
  wrAddrNext : Switch  Criteria=u2 ~= 0  Threshold=double(0)  OutDataTypeStr=fixdt(0, 10, 0)  SampleTime=2.77039007092199e-06  SaturateOnIntegerOverflow=off  InputSameDT=off
  wrAddrPlusOne : Sum  OutDataTypeStr=fixdt(0, 10, 0)  SampleTime=2.77039007092199e-06
  wrEn : Logic  Operator=OR  AllPortsSameDT=off  OutDataTypeStr=boolean  SampleTime=2.77039007092199e-06
  zero : Constant  Value=0  OutDataTypeStr=fixdt(0, 10, 0)  SampleTime=2.77039007092199e-06
  sample : Outport  OutDataTypeStr=single  SampleTime=2.77039007092199e-06
  onEndVals : Outport  Port=2  OutDataTypeStr=boolean  SampleTime=2.77039007092199e-06
  wires:
  sample_in/1 -> ram_generic/1
  onEndVals_in/1 -> endValsLoad/1, wrEn/2
  valid/1 -> wrEn/1
  isLastSample/1 -> endValsLoad/2
  wrEn/1 -> rdEn/1, wrAddrNext/2, wrAddr/1, ram_generic/3
  wrAddr/1 -> wrAddrNext/3, wrAddrIsMax/1, wrAddrPlusOne/1, ram_generic/2
  one/1 -> wrAddrPlusOne/2
  wrAddrPlusOne/1 -> wrAddrIncr/3
  zero/1 -> wrAddrIncr/1
  wrAddrIsMax/1 -> wrAddrIncr/2
  wrAddrIncr/1 -> wrAddrNext/1
  wrAddrNext/1 -> rdAddr/2
  endValsCount/1 -> rdAddrLoad/1, onEndVals1/1
  onEndVals1/1 -> onEndVals/1, rdEn/2, endValsCount/3
  endValsLoad/1 -> endValsCount/1
  endValsCount_loadValue/1 -> endValsCount/2
  rdAddrLoad/1 -> rdAddr/1
  rdEn/1 -> enb/1, rdAddr/3
  rdAddr/1 -> ram_generic/4
  ram_generic/1 -> sample1/1
  enb/1 -> sample1/2
  sample1/1 -> sample/1, sample_hold/1
  sample_hold/1 -> sample1/3

== system gm_gaussianFilter/gaussianFilter/streaming_matrix_partition/frameBasedGaussianFilter/ImageIn_NeighborhoodCreator/NeighborhoodCreator_3x3/row2_col1 ==
  sample_in : Inport  OutDataTypeStr=single  SampleTime=2.77039007092199e-06
  onEndVals_in : Inport  Port=2  OutDataTypeStr=boolean  SampleTime=2.77039007092199e-06
  valid : Inport  Port=3  OutDataTypeStr=boolean  SampleTime=2.77039007092199e-06
  isLastSample : Inport  Port=4  OutDataTypeStr=boolean  SampleTime=2.77039007092199e-06
  enb : Logic  Operator=OR  AllPortsSameDT=off  OutDataTypeStr=boolean  SampleTime=2.77039007092199e-06
  onEndVals1 : Logic  Operator=OR  AllPortsSameDT=off  OutDataTypeStr=boolean  SampleTime=2.77039007092199e-06
  onEndVals_delay : Delay  DelayLength=double(1)  InitialCondition=0  SampleTime=2.77039007092199e-06
  sample_delayed : Delay  DelayLength=double(1)  InitialCondition=double(0)  ShowEnablePort=on
      settings: InputPortMap=u0,e6
  sample : Outport  OutDataTypeStr=single  SampleTime=2.77039007092199e-06
  onEndVals : Outport  Port=2  OutDataTypeStr=boolean  SampleTime=2.77039007092199e-06
  wires:
  sample_in/1 -> sample_delayed/1
  onEndVals_in/1 -> onEndVals1/1
  valid/1 -> enb/1
  isLastSample/1 -> onEndVals1/2
  onEndVals1/1 -> onEndVals_delay/1
  onEndVals_delay/1 -> onEndVals/1, enb/2
  enb/1 -> sample_delayed/2
  sample_delayed/1 -> sample/1

== system gm_gaussianFilter/gaussianFilter/streaming_matrix_partition/frameBasedGaussianFilter/ImageIn_NeighborhoodCreator/NeighborhoodCreator_3x3/row2_col2 ==
  sample_in : Inport  OutDataTypeStr=single  SampleTime=2.77039007092199e-06
  onEndVals_in : Inport  Port=2  OutDataTypeStr=boolean  SampleTime=2.77039007092199e-06
  valid : Inport  Port=3  OutDataTypeStr=boolean  SampleTime=2.77039007092199e-06
  isLastSample : Inport  Port=4  OutDataTypeStr=boolean  SampleTime=2.77039007092199e-06
  enb : Logic  Operator=OR  AllPortsSameDT=off  OutDataTypeStr=boolean  SampleTime=2.77039007092199e-06
  onEndVals1 : Logic  Operator=OR  AllPortsSameDT=off  OutDataTypeStr=boolean  SampleTime=2.77039007092199e-06
  onEndVals_delay : Delay  DelayLength=double(1)  InitialCondition=0  SampleTime=2.77039007092199e-06
  sample_delayed : Delay  DelayLength=double(1)  InitialCondition=double(0)  ShowEnablePort=on
      settings: InputPortMap=u0,e6
  sample : Outport  OutDataTypeStr=single  SampleTime=2.77039007092199e-06
  onEndVals : Outport  Port=2  OutDataTypeStr=boolean  SampleTime=2.77039007092199e-06
  wires:
  sample_in/1 -> sample_delayed/1
  onEndVals_in/1 -> onEndVals1/1
  valid/1 -> enb/1
  isLastSample/1 -> onEndVals1/2
  onEndVals1/1 -> onEndVals_delay/1
  onEndVals_delay/1 -> onEndVals/1, enb/2
  enb/1 -> sample_delayed/2
  sample_delayed/1 -> sample/1

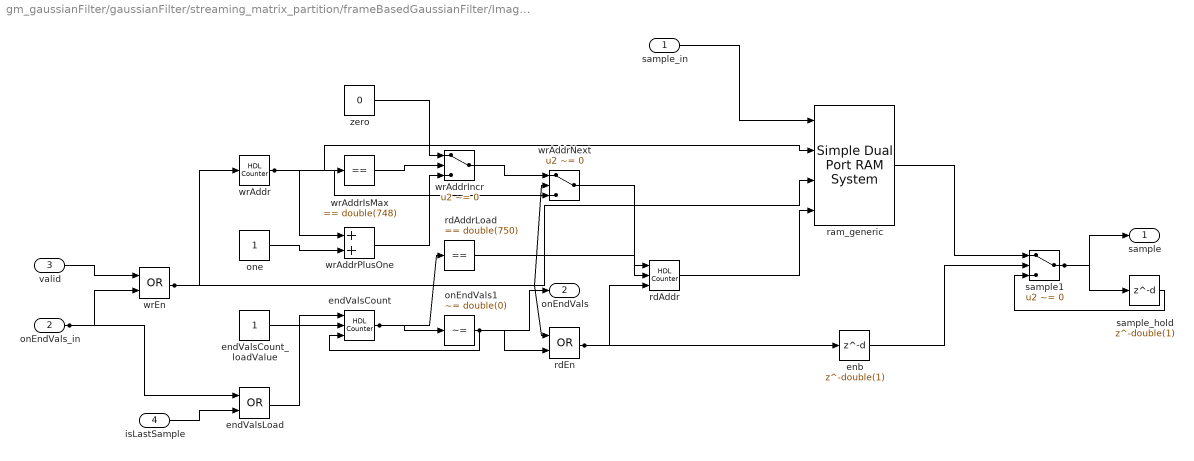
== system gm_gaussianFilter/gaussianFilter/streaming_matrix_partition/frameBasedGaussianFilter/ImageIn_NeighborhoodCreator/NeighborhoodCreator_3x3/row2_linebuffer ==
  sample_in : Inport  OutDataTypeStr=single  SampleTime=2.77039007092199e-06
  onEndVals_in : Inport  Port=2  OutDataTypeStr=boolean  SampleTime=2.77039007092199e-06
  valid : Inport  Port=3  OutDataTypeStr=boolean  SampleTime=2.77039007092199e-06
  isLastSample : Inport  Port=4  OutDataTypeStr=boolean  SampleTime=2.77039007092199e-06
  enb : Delay  DelayLength=double(1)  InitialCondition=0  SampleTime=2.77039007092199e-06
  endValsCount : hdlsllib/Sources/HDL Counter  CountType=Count limited  CountInit=double(0)  CountStep=double(1)  CountMax=double(750)  CountFromType=Initial value  CountFrom=double(0)  CountResetPort=off  CountLoadPort=on  CountEnbPort=on  CountDirPort=off  CountHitOutputPort=off  CountDataType=Unsigned  CountWordLen=10  CountFracLen=0  CountSampTime=2.77039007092199e-06
  endValsCount_loadValue : Constant  OutDataTypeStr=fixdt(0, 10, 0)  SampleTime=2.77039007092199e-06
  endValsLoad : Logic  Operator=OR  AllPortsSameDT=off  OutDataTypeStr=boolean  SampleTime=2.77039007092199e-06
  onEndVals1 : simulink/Logic and Bit Operations/Compare To Constant  relop=~=  const=double(0)  OutDataTypeStr=boolean
  one : Constant  OutDataTypeStr=fixdt(0, 10, 0)  SampleTime=2.77039007092199e-06
  ram_generic : hdlsllib/HDL RAMs/Simple Dual Port RAM System  RAMType=Simple dual port  AsyncRead=off  WriteOutputValue=New data  RAMInitialValue=0  allowBusInputs=off  WritesHaveOutput=on  NumReads=0  NumWrites=1  SimulateUsing=Code generation
  rdAddr : hdlsllib/Sources/HDL Counter  CountType=Count limited  CountInit=double(0)  CountStep=double(1)  CountMax=double(748)  CountFromType=Initial value  CountFrom=double(0)  CountResetPort=off  CountLoadPort=on  CountEnbPort=on  CountDirPort=off  CountHitOutputPort=off  CountDataType=Unsigned  CountWordLen=10  CountFracLen=0  CountSampTime=2.77039007092199e-06
  rdAddrLoad : simulink/Logic and Bit Operations/Compare To Constant  relop===  const=double(750)  OutDataTypeStr=boolean
  rdEn : Logic  Operator=OR  AllPortsSameDT=off  OutDataTypeStr=boolean  SampleTime=2.77039007092199e-06
  sample1 : Switch  Criteria=u2 ~= 0  Threshold=double(0)  OutDataTypeStr=single  SampleTime=2.77039007092199e-06  SaturateOnIntegerOverflow=off  InputSameDT=off
  sample_hold : Delay  DelayLength=double(1)  InitialCondition=0  SampleTime=2.77039007092199e-06
  wrAddr : hdlsllib/Sources/HDL Counter  CountType=Count limited  CountInit=double(0)  CountStep=double(1)  CountMax=double(748)  CountFromType=Initial value  CountFrom=double(0)  CountResetPort=off  CountLoadPort=off  CountEnbPort=on  CountDirPort=off  CountHitOutputPort=off  CountDataType=Unsigned  CountWordLen=10  CountFracLen=0  CountSampTime=2.77039007092199e-06
  wrAddrIncr : Switch  Criteria=u2 ~= 0  Threshold=double(0)  OutDataTypeStr=fixdt(0, 10, 0)  SampleTime=2.77039007092199e-06  SaturateOnIntegerOverflow=off  InputSameDT=off
  wrAddrIsMax : simulink/Logic and Bit Operations/Compare To Constant  relop===  const=double(748)  OutDataTypeStr=boolean
  wrAddrNext : Switch  Criteria=u2 ~= 0  Threshold=double(0)  OutDataTypeStr=fixdt(0, 10, 0)  SampleTime=2.77039007092199e-06  SaturateOnIntegerOverflow=off  InputSameDT=off
  wrAddrPlusOne : Sum  OutDataTypeStr=fixdt(0, 10, 0)  SampleTime=2.77039007092199e-06
  wrEn : Logic  Operator=OR  AllPortsSameDT=off  OutDataTypeStr=boolean  SampleTime=2.77039007092199e-06
  zero : Constant  Value=0  OutDataTypeStr=fixdt(0, 10, 0)  SampleTime=2.77039007092199e-06
  sample : Outport  OutDataTypeStr=single  SampleTime=2.77039007092199e-06
  onEndVals : Outport  Port=2  OutDataTypeStr=boolean  SampleTime=2.77039007092199e-06
  wires:
  sample_in/1 -> ram_generic/1
  onEndVals_in/1 -> endValsLoad/1, wrEn/2
  valid/1 -> wrEn/1
  isLastSample/1 -> endValsLoad/2
  wrEn/1 -> rdEn/1, wrAddrNext/2, wrAddr/1, ram_generic/3
  wrAddr/1 -> wrAddrNext/3, wrAddrIsMax/1, wrAddrPlusOne/1, ram_generic/2
  one/1 -> wrAddrPlusOne/2
  wrAddrPlusOne/1 -> wrAddrIncr/3
  zero/1 -> wrAddrIncr/1
  wrAddrIsMax/1 -> wrAddrIncr/2
  wrAddrIncr/1 -> wrAddrNext/1
  wrAddrNext/1 -> rdAddr/2
  endValsCount/1 -> rdAddrLoad/1, onEndVals1/1
  onEndVals1/1 -> onEndVals/1, rdEn/2, endValsCount/3
  endValsLoad/1 -> endValsCount/1
  endValsCount_loadValue/1 -> endValsCount/2
  rdAddrLoad/1 -> rdAddr/1
  rdEn/1 -> enb/1, rdAddr/3
  rdAddr/1 -> ram_generic/4
  ram_generic/1 -> sample1/1
  enb/1 -> sample1/2
  sample1/1 -> sample/1, sample_hold/1
  sample_hold/1 -> sample1/3

== system gm_gaussianFilter/gaussianFilter/streaming_matrix_partition/frameBasedGaussianFilter/ImageIn_NeighborhoodCreator/NeighborhoodCreator_3x3/row3_col1 ==
  sample_in : Inport  OutDataTypeStr=single  SampleTime=2.77039007092199e-06
  onEndVals_in : Inport  Port=2  OutDataTypeStr=boolean  SampleTime=2.77039007092199e-06
  valid : Inport  Port=3  OutDataTypeStr=boolean  SampleTime=2.77039007092199e-06
  isLastSample : Inport  Port=4  OutDataTypeStr=boolean  SampleTime=2.77039007092199e-06
  enb : Logic  Operator=OR  AllPortsSameDT=off  OutDataTypeStr=boolean  SampleTime=2.77039007092199e-06
  onEndVals1 : Logic  Operator=OR  AllPortsSameDT=off  OutDataTypeStr=boolean  SampleTime=2.77039007092199e-06
  onEndVals_delay : Delay  DelayLength=double(1)  InitialCondition=0  SampleTime=2.77039007092199e-06
  sample_delayed : Delay  DelayLength=double(1)  InitialCondition=double(0)  ShowEnablePort=on
      settings: InputPortMap=u0,e6
  sample : Outport  OutDataTypeStr=single  SampleTime=2.77039007092199e-06
  onEndVals : Outport  Port=2  OutDataTypeStr=boolean  SampleTime=2.77039007092199e-06
  wires:
  sample_in/1 -> sample_delayed/1
  onEndVals_in/1 -> onEndVals1/1
  valid/1 -> enb/1
  isLastSample/1 -> onEndVals1/2
  onEndVals1/1 -> onEndVals_delay/1
  onEndVals_delay/1 -> onEndVals/1, enb/2
  enb/1 -> sample_delayed/2
  sample_delayed/1 -> sample/1

== system gm_gaussianFilter/gaussianFilter/streaming_matrix_partition/frameBasedGaussianFilter/ImageIn_NeighborhoodCreator/NeighborhoodCreator_3x3/row3_col2 ==
  sample_in : Inport  OutDataTypeStr=single  SampleTime=2.77039007092199e-06
  onEndVals_in : Inport  Port=2  OutDataTypeStr=boolean  SampleTime=2.77039007092199e-06
  valid : Inport  Port=3  OutDataTypeStr=boolean  SampleTime=2.77039007092199e-06
  isLastSample : Inport  Port=4  OutDataTypeStr=boolean  SampleTime=2.77039007092199e-06
  enb : Logic  Operator=OR  AllPortsSameDT=off  OutDataTypeStr=boolean  SampleTime=2.77039007092199e-06
  onEndVals1 : Logic  Operator=OR  AllPortsSameDT=off  OutDataTypeStr=boolean  SampleTime=2.77039007092199e-06
  onEndVals_delay : Delay  DelayLength=double(1)  InitialCondition=0  SampleTime=2.77039007092199e-06
  sample_delayed : Delay  DelayLength=double(1)  InitialCondition=double(0)  ShowEnablePort=on
      settings: InputPortMap=u0,e6
  sample : Outport  OutDataTypeStr=single  SampleTime=2.77039007092199e-06
  onEndVals : Outport  Port=2  OutDataTypeStr=boolean  SampleTime=2.77039007092199e-06
  wires:
  sample_in/1 -> sample_delayed/1
  onEndVals_in/1 -> onEndVals1/1
  valid/1 -> enb/1
  isLastSample/1 -> onEndVals1/2
  onEndVals1/1 -> onEndVals_delay/1
  onEndVals_delay/1 -> onEndVals/1, enb/2
  enb/1 -> sample_delayed/2
  sample_delayed/1 -> sample/1

== matlab function gm_gaussianFilter/Input streaming/coeffs_tb ==
  data: coeffs_in input; coeffs_out output; validIn input
function coeffs_out = coeffs_tb(coeffs_in, validIn)

persistent samples validCount;

if isempty(validCount)
    samples = cell(1, 0);
    validCount = 360960;
end

samples{end+1} = coeffs_in;
coeffs_out = zeros(size(coeffs_in), 'like', coeffs_in);

if validIn
    if validCount == 360960
        validCount = 0;
        coeffs_out = samples{1};
    end

    validCount = validCount + 1;
    samples(1) = [];
end

== matlab function gm_gaussianFilter/Input streaming/imageIn_tb ==
  data: imageIn_sample input; imageIn_out_sample output; imageIn_ready input; imageIn_valid output; numLowValidCycles parameter; numHighValidCycles parameter; toggleValid parameter
function [imageIn_out_sample, imageIn_valid] = imageIn_tb(imageIn_sample, imageIn_ready, numLowValidCycles, numHighValidCycles, toggleValid)

persistent samples validCount sendValid;

if isempty(validCount)
    samples = cell(1, 0);
    validCount = 0;
    sendValid = true;
end

samples{end+1} = imageIn_sample;

if sendValid
    imageIn_valid = true;
    imageIn_out_sample = samples{1};

    if imageIn_ready
        samples(1) = [];

        if toggleValid
            validCount = validCount + 1;

            if validCount >= numHighValidCycles
                validCount = 0;
                sendValid = false;
            end
        end
    end
else
    imageIn_valid = false;
    imageIn_out_sample = zeros(size(samples{1}), 'like', samples{1});

    if imageIn_ready
        validCount = validCount + 1;

        if validCount >= numLowValidCycles
            validCount = 0;
            sendValid = true;
        end
    end
end

== matlab function gm_gaussianFilter/Input streaming/imageOut_ready_tb ==
  data: imageOut_ready output; numLowReadyCycles parameter; numHighReadyCycles parameter; toggleReady parameter
function imageOut_ready = imageOut_ready_tb(numLowReadyCycles, numHighReadyCycles, toggleReady)

persistent readyCount sendReady;

if isempty(readyCount)
    readyCount = 0;
    sendReady = true;
end

if sendReady
    imageOut_ready = true;

    if toggleReady
        readyCount = readyCount + 1;

        if readyCount >= numHighReadyCycles
            readyCount = 0;
            sendReady = false;
        end
    end
else
    imageOut_ready = false;

    readyCount = readyCount + 1;
    if readyCount >= numLowReadyCycles
        readyCount = 0;
        sendReady = true;
    end
end
